simulink model "PID_SMC_for_Hexa_rotor"  (R2021a)
settings: Solver=VariableStepAuto  StartTime=0.0  StopTime=T_s+30  RelTol=1e-3
StartFcn:
  | run('Linearized_model.m')
values from neighbouring files (symbols this model uses):
  a_x = x(1,1:(length(x)-1))    [Linearized_model.m]    (also in Linearized_model_motor_dynamics.m)
  a_y = y(1,1:(length(y)-1))    [Linearized_model.m]    (also in Linearized_model_motor_dynamics.m)
  a_z = z(1,1:(length(z)-1))    [Linearized_model.m]    (also in Linearized_model_motor_dynamics.m)
  b_x = x(1,2:length(x))    [Linearized_model.m]    (also in Linearized_model_motor_dynamics.m)
  b_y = y(1,2:length(y))    [Linearized_model.m]    (also in Linearized_model_motor_dynamics.m)
  b_z = z(1,2:length(z))    [Linearized_model.m]    (also in Linearized_model_motor_dynamics.m)
  T_r = zeros(1, length(T))    [Linearized_model.m]    (also in Linearized_model_motor_dynamics.m)
  T_s = sum(T)    [Linearized_model.m]    (also in Linearized_model_motor_dynamics.m)
undefined symbols (not defined in the file or in its folder): a_phi, a_si, a_theta, b_phi, b_si, b_theta
libraries: sharedtransform x1, uavutilslib x1
settings Model: Creator=Traveler  LastModifiedBy=Traveler

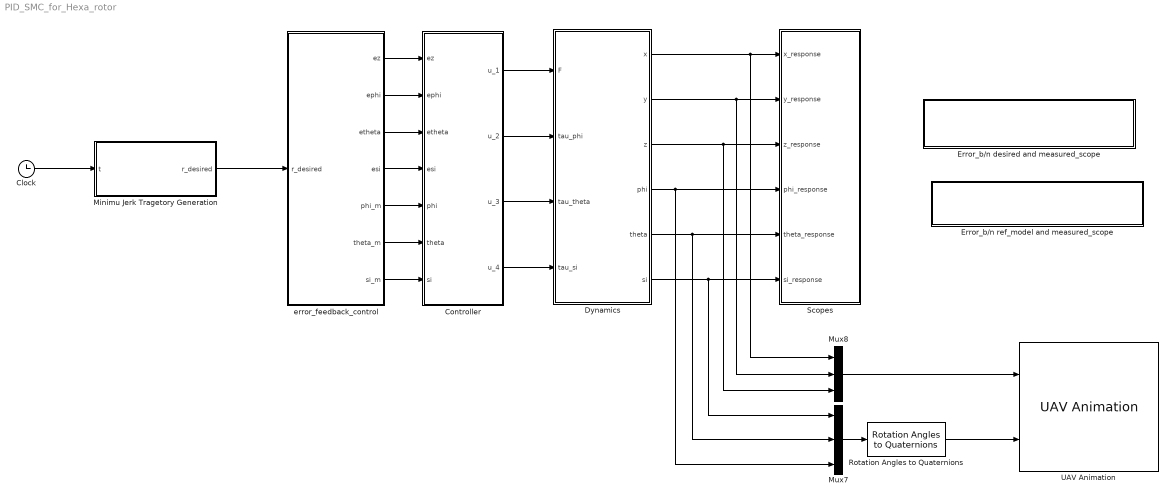
== system PID_SMC_for_Hexa_rotor ==
  Clock : Clock
  Controller : Subsystem
  Dynamics : Subsystem
  Error_b/n desired and measured_scope : Subsystem
  Error_b/n ref_model and measured_scope : Subsystem
  Minimu Jerk Tragetory Generation : Subsystem
  Mux7 : Mux  Inputs=3
  Mux8 : Mux  Inputs=3
  Rotation Angles to Quaternions : sharedtransform/Rotation Angles to Quaternions  rotationOrder=ZYX  aMode=aMode
      settings: SourceProductBaseCode=AE,PW,DR,MT,UV,VE
  Scopes : Subsystem
  UAV Animation : uavutilslib/UAV Animation  UAVType=Multirotor  UAVSize=0.1  InertialZDirection=Up  SampleTime=0.1
      settings: SourceProductBaseCode=UV
  error_feedback_control : Subsystem
  wires:
  error_feedback_control/1(ez) -> Controller/1(ez)
  error_feedback_control/7(si_m) -> Controller/7(si)
  Controller/1(u_1) -> Dynamics/1(F)
  error_feedback_control/2(ephi) -> Controller/2(ephi)
  error_feedback_control/6(theta_m) -> Controller/6(theta)
  error_feedback_control/4(esi) -> Controller/4(esi)
  Clock/1 -> Minimu Jerk Tragetory Generation/1(t)
  error_feedback_control/3(etheta) -> Controller/3(etheta)
  error_feedback_control/5(phi_m) -> Controller/5(phi)
  Controller/2(u_2) -> Dynamics/2(tau_phi)
  Controller/4(u_4) -> Dynamics/4(tau_si)
  Controller/3(u_3) -> Dynamics/3(tau_theta)
  Minimu Jerk Tragetory Generation/1(r_desired) -> error_feedback_control/1(r_desired)
  Rotation Angles to Quaternions/1 -> UAV Animation/2
  Dynamics/2(y) -> Mux8/2, Scopes/2(y_response)
  Mux7/1 -> Rotation Angles to Quaternions/1
  Dynamics/6(si) -> Mux7/1, Scopes/6(si_response)
  Dynamics/1(x) -> Mux8/1, Scopes/1(x_response)
  Dynamics/5(theta) -> Mux7/2, Scopes/5(theta_response)
  Dynamics/3(z) -> Mux8/3, Scopes/3(z_response)
  Dynamics/4(phi) -> Mux7/3, Scopes/4(phi_response)
  Mux8/1 -> UAV Animation/1

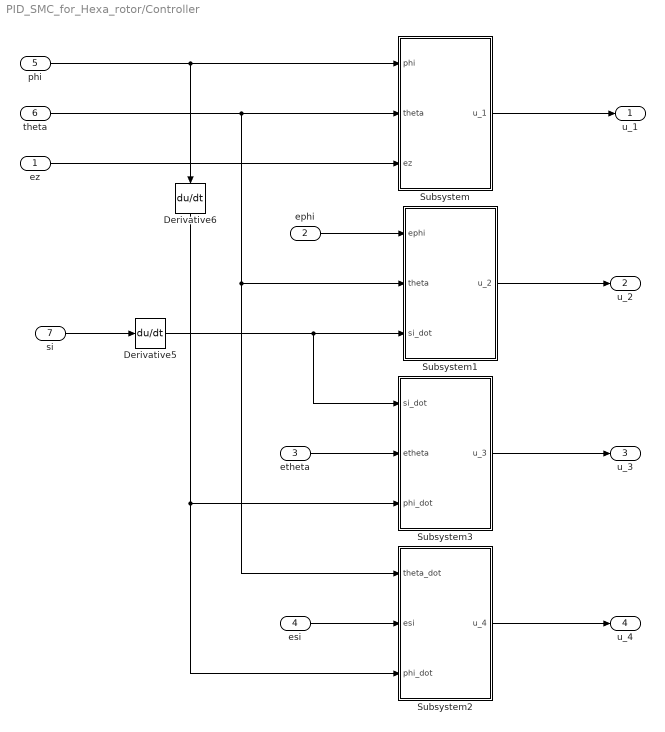
== system PID_SMC_for_Hexa_rotor/Controller ==
  ez : Inport
  ephi : Inport  Port=2
  etheta : Inport  Port=3
  esi : Inport  Port=4
  phi : Inport  Port=5
  theta : Inport  Port=6
  si : Inport  Port=7
  Derivative5 : Derivative
  Derivative6 : Derivative
  Subsystem : Subsystem
  Subsystem1 : Subsystem
  Subsystem2 : Subsystem
  Subsystem3 : Subsystem
  u_1 : Outport
  u_2 : Outport  Port=2
  u_3 : Outport  Port=3
  u_4 : Outport  Port=4
  wires:
  phi/1 -> Derivative6/1, Subsystem/1(phi)
  theta/1 -> Subsystem2/1(theta_dot), Subsystem1/2(theta), Subsystem/2(theta)
  Derivative5/1 -> Subsystem1/3(si_dot), Subsystem3/1(si_dot)
  Derivative6/1 -> Subsystem2/3(phi_dot), Subsystem3/3(phi_dot)
  si/1 -> Derivative5/1
  ez/1 -> Subsystem/3(ez)
  Subsystem/1(u_1) -> u_1/1
  ephi/1 -> Subsystem1/1(ephi)
  Subsystem1/1(u_2) -> u_2/1
  esi/1 -> Subsystem2/2(esi)
  Subsystem2/1(u_4) -> u_4/1
  etheta/1 -> Subsystem3/2(etheta)
  Subsystem3/1(u_3) -> u_3/1

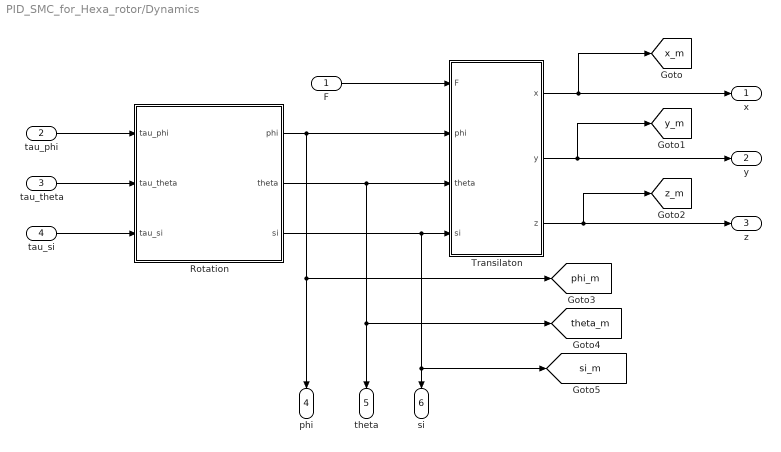
== system PID_SMC_for_Hexa_rotor/Dynamics ==
  F : Inport
  tau_phi : Inport  Port=2
  tau_theta : Inport  Port=3
  tau_si : Inport  Port=4
  Rotation : Subsystem
  Transilaton : Subsystem
  x : Outport
  y : Outport  Port=2
  z : Outport  Port=3
  phi : Outport  Port=4
  theta : Outport  Port=5
  si : Outport  Port=6
  tag scope: phi_m=global, si_m=global, theta_m=global, x_m=global, y_m=global, z_m=global
  wires:
  Transilaton/2(y) -> [y_m], y/1
  Transilaton/1(x) -> [x_m], x/1
  Transilaton/3(z) -> [z_m], z/1
  Rotation/1(phi) -> Transilaton/2(phi), phi/1, [phi_m]
  Rotation/2(theta) -> Transilaton/3(theta), theta/1, [theta_m]
  Rotation/3(si) -> Transilaton/4(si), [si_m], si/1
  tau_phi/1 -> Rotation/1(tau_phi)
  tau_theta/1 -> Rotation/2(tau_theta)
  tau_si/1 -> Rotation/3(tau_si)
  F/1 -> Transilaton/1(F)

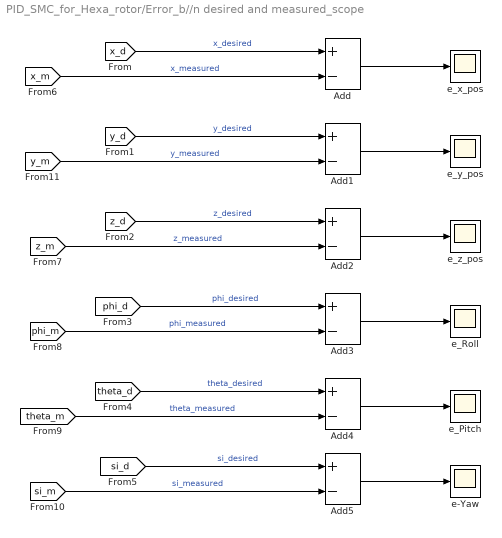
== system PID_SMC_for_Hexa_rotor/Error_b//n desired and measured_scope ==
  Add{,1..5} (6 alike) : Sum  Inputs=+-
  e-Yaw : Scope
  e_Pitch : Scope
  e_Roll : Scope
  e_x_pos : Scope
  e_y_pos : Scope
  e_z_pos : Scope
  wires:
  [x_m] -> Add/2  "x_measured"
  Add/1 -> e_x_pos/1
  [x_d] -> Add/1  "x_desired"
  [y_d] -> Add1/1  "y_desired"
  Add1/1 -> e_y_pos/1
  [z_m] -> Add2/2  "z_measured"
  [z_d] -> Add2/1  "z_desired"
  [phi_d] -> Add3/1  "phi_desired"
  [phi_m] -> Add3/2  "phi_measured"
  [theta_m] -> Add4/2  "theta_measured"
  [theta_d] -> Add4/1  "theta_desired"
  [si_d] -> Add5/1  "si_desired"
  [si_m] -> Add5/2  "si_measured"
  Add2/1 -> e_z_pos/1
  [y_m] -> Add1/2  "y_measured"
  Add5/1 -> e-Yaw/1
  Add3/1 -> e_Roll/1
  Add4/1 -> e_Pitch/1

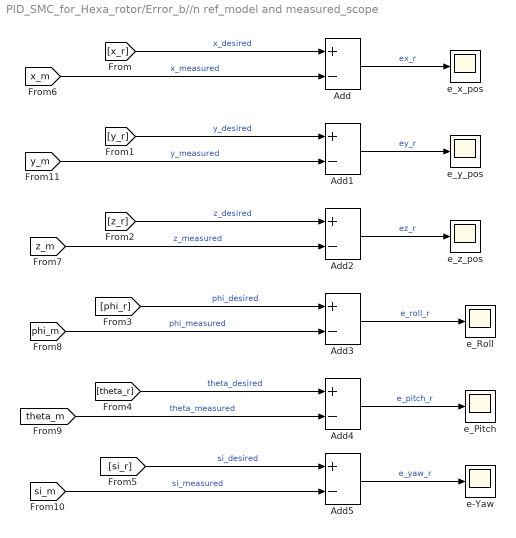
== system PID_SMC_for_Hexa_rotor/Error_b//n ref_model and measured_scope ==
  Add{,1..5} (6 alike) : Sum  Inputs=+-
  e-Yaw : Scope
  e_Pitch : Scope
  e_Roll : Scope
  e_x_pos : Scope
  e_y_pos : Scope
  e_z_pos : Scope
  wires:
  Add4/1 -> e_Pitch/1  "e_pitch_r"
  Add3/1 -> e_Roll/1  "e_roll_r"
  Add5/1 -> e-Yaw/1  "e_yaw_r"
  [y_m] -> Add1/2  "y_measured"
  Add2/1 -> e_z_pos/1  "ez_r"
  [si_m] -> Add5/2  "si_measured"
  [si_r] -> Add5/1  "si_desired"
  [theta_r] -> Add4/1  "theta_desired"
  [theta_m] -> Add4/2  "theta_measured"
  [phi_m] -> Add3/2  "phi_measured"
  [phi_r] -> Add3/1  "phi_desired"
  [z_r] -> Add2/1  "z_desired"
  [z_m] -> Add2/2  "z_measured"
  Add1/1 -> e_y_pos/1  "ey_r"
  [y_r] -> Add1/1  "y_desired"
  [x_r] -> Add/1  "x_desired"
  Add/1 -> e_x_pos/1  "ex_r"
  [x_m] -> Add/2  "x_measured"

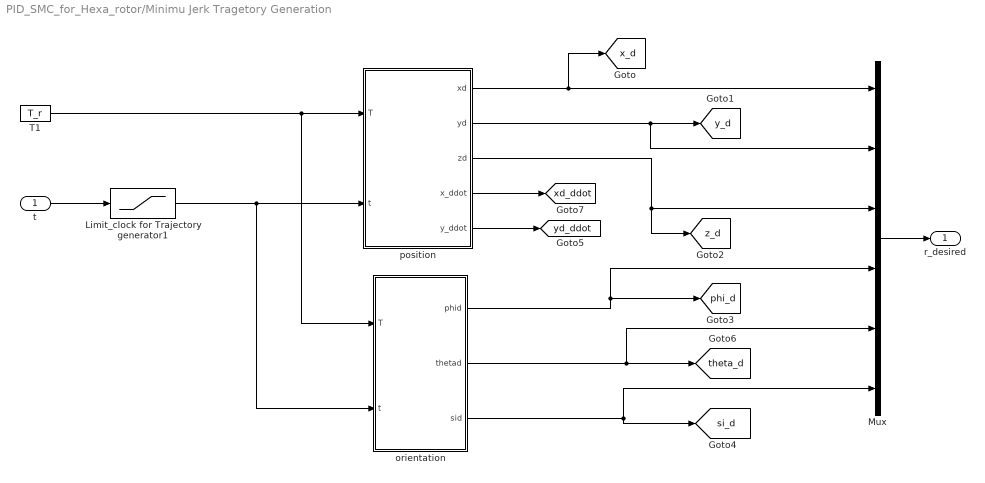
== system PID_SMC_for_Hexa_rotor/Minimu Jerk Tragetory Generation ==
  t : Inport
  Limit_clock for Trajectory generator1 : Saturate  UpperLimit=T_s  LowerLimit=0
  Mux : Mux  Inputs=6
  T1 : Constant  Value=T_r
  orientation : Subsystem
  position : Subsystem
  r_desired : Outport
  tag scope: phi_d=global, si_d=global, theta_d=global, x_d=global, xd_ddot=global, y_d=global, yd_ddot=global, z_d=global
  wires:
  Mux/1 -> r_desired/1
  orientation/1(phid) -> Mux/4, [phi_d]
  orientation/3(sid) -> [si_d], Mux/6
  position/4(x_ddot) -> [xd_ddot]
  position/1(xd) -> Mux/1, [x_d]
  position/3(zd) -> Mux/3, [z_d]
  Limit_clock for Trajectory generator1/1 -> position/2(t), orientation/2(t)
  T1/1 -> position/1(T), orientation/1(T)
  position/5(y_ddot) -> [yd_ddot]
  t/1 -> Limit_clock for Trajectory generator1/1
  orientation/2(thetad) -> Mux/5, [theta_d]
  position/2(yd) -> Mux/2, [y_d]

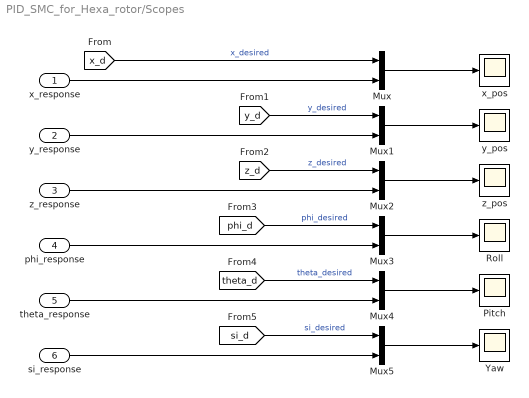
== system PID_SMC_for_Hexa_rotor/Scopes ==
  x_response : Inport
  y_response : Inport  Port=2
  z_response : Inport  Port=3
  phi_response : Inport  Port=4
  theta_response : Inport  Port=5
  si_response : Inport  Port=6
  Mux{,1..5} (6 alike) : Mux  Inputs=2
  Pitch : Scope
  Roll : Scope
  Yaw : Scope
  x_pos : Scope
  y_pos : Scope
  z_pos : Scope
  wires:
  [x_d] -> Mux/1  "x_desired"
  Mux4/1 -> Pitch/1
  [phi_d] -> Mux3/1  "phi_desired"
  Mux2/1 -> z_pos/1
  [si_d] -> Mux5/1  "si_desired"
  [y_d] -> Mux1/1  "y_desired"
  [theta_d] -> Mux4/1  "theta_desired"
  Mux5/1 -> Yaw/1
  Mux/1 -> x_pos/1
  [z_d] -> Mux2/1  "z_desired"
  Mux3/1 -> Roll/1
  y_response/1 -> Mux1/2
  Mux1/1 -> y_pos/1
  theta_response/1 -> Mux4/2
  z_response/1 -> Mux2/2
  phi_response/1 -> Mux3/2
  si_response/1 -> Mux5/2
  x_response/1 -> Mux/2

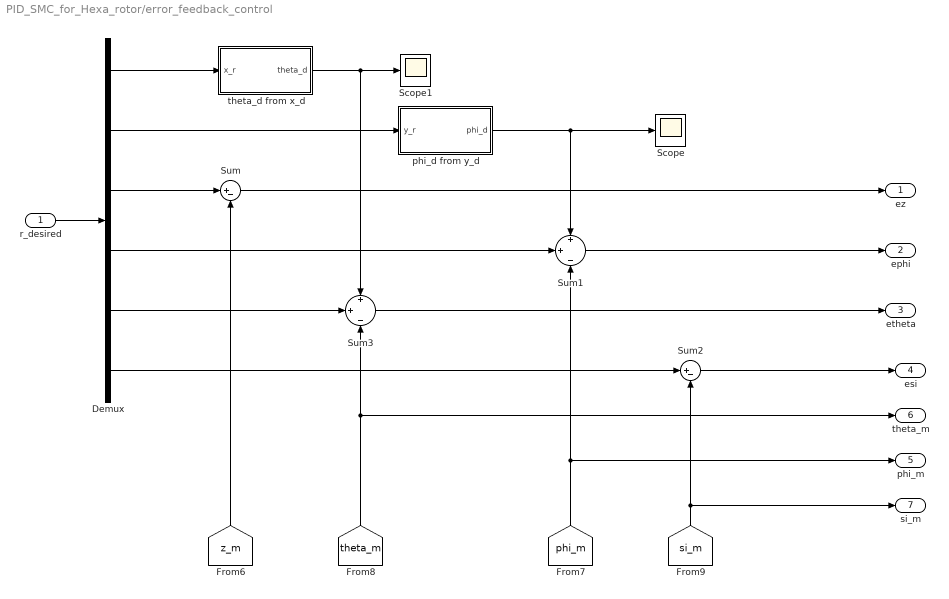
== system PID_SMC_for_Hexa_rotor/error_feedback_control ==
  r_desired : Inport
  Demux : Demux  Outputs=6
  Scope : Scope
  Scope1 : Scope
  Sum : Sum  Inputs=|+-
  Sum1 : Sum  Inputs=+|+|-
  Sum2 : Sum  Inputs=|+-
  Sum3 : Sum  Inputs=+|+|-
  phi_d from y_d : Subsystem
  theta_d from x_d : Subsystem
  ez : Outport
  ephi : Outport  Port=2
  etheta : Outport  Port=3
  esi : Outport  Port=4
  phi_m : Outport  Port=5
  theta_m : Outport  Port=6
  si_m : Outport  Port=7
  wires:
  [theta_m] -> Sum3/3, theta_m/1
  Demux/5 -> Sum3/2
  [phi_m] -> Sum1/3, phi_m/1
  [si_m] -> si_m/1, Sum2/2
  Demux/6 -> Sum2/1
  [z_m] -> Sum/2
  Demux/3 -> Sum/1
  Sum1/1 -> ephi/1
  Sum3/1 -> etheta/1
  Sum/1 -> ez/1
  Sum2/1 -> esi/1
  r_desired/1 -> Demux/1
  Demux/1 -> theta_d from x_d/1(x_r)
  Demux/2 -> phi_d from y_d/1(y_r)
  Demux/4 -> Sum1/2
  phi_d from y_d/1(phi_d) -> Scope/1, Sum1/1
  theta_d from x_d/1(theta_d) -> Sum3/1, Scope1/1

== system PID_SMC_for_Hexa_rotor/Controller/Subsystem ==
  phi : Inport
  theta : Inport  Port=2
  ez : Inport  Port=3
  Derivative : Derivative
  Integrator : Integrator
  Integrator4 : Integrator
  Sliding Mode controller : MATLAB Function  TreatAsAtomicUnit=on
  u_1 : Outport
  wires:
  ez/1 -> Integrator4/1, Derivative/1, Sliding Mode controller/3(ez)
  Integrator4/1 -> Sliding Mode controller/5(ez_int)
  Sliding Mode controller/2(del_hat_dot) -> Integrator/1
  Derivative/1 -> Sliding Mode controller/4(ez_dot)
  Integrator/1 -> Sliding Mode controller/6(del_hat)
  Sliding Mode controller/1(u_1) -> u_1/1
  phi/1 -> Sliding Mode controller/1(phi)
  theta/1 -> Sliding Mode controller/2(theta)

== system PID_SMC_for_Hexa_rotor/Controller/Subsystem1 ==
  ephi : Inport
  theta : Inport  Port=2
  si_dot : Inport  Port=3
  Derivative1 : Derivative
  Derivative4 : Derivative
  Integrator3 : Integrator
  Integrator5 : Integrator
  Sliding Mode controller1 : MATLAB Function  TreatAsAtomicUnit=on
  u_2 : Outport
  wires:
  Sliding Mode controller1/2(del_hat_dot) -> Integrator3/1
  ephi/1 -> Integrator5/1, Derivative1/1, Sliding Mode controller1/1(ephi)
  theta/1 -> Derivative4/1
  Derivative1/1 -> Sliding Mode controller1/2(ephi_dot)
  Sliding Mode controller1/1(u_2) -> u_2/1
  Derivative4/1 -> Sliding Mode controller1/4(theta_dot)
  Integrator3/1 -> Sliding Mode controller1/6(del_hat)
  Integrator5/1 -> Sliding Mode controller1/3(ephi_int)
  si_dot/1 -> Sliding Mode controller1/5(si_dot)

== system PID_SMC_for_Hexa_rotor/Controller/Subsystem2 ==
  theta_dot : Inport
  esi : Inport  Port=2
  phi_dot : Inport  Port=3
  Derivative3 : Derivative
  Integrator2 : Integrator
  Integrator7 : Integrator
  Sliding Mode controller3 : MATLAB Function  TreatAsAtomicUnit=on
  u_4 : Outport
  wires:
  theta_dot/1 -> Sliding Mode controller3/4(theta_dot)
  esi/1 -> Sliding Mode controller3/1(esi), Integrator7/1, Derivative3/1
  Derivative3/1 -> Sliding Mode controller3/2(esi_dot)
  Integrator2/1 -> Sliding Mode controller3/6(del_hat)
  Integrator7/1 -> Sliding Mode controller3/3(esi_int)
  Sliding Mode controller3/2(del_hat_dot) -> Integrator2/1
  Sliding Mode controller3/1(u_4) -> u_4/1
  phi_dot/1 -> Sliding Mode controller3/5(phi_dot)

== system PID_SMC_for_Hexa_rotor/Controller/Subsystem3 ==
  si_dot : Inport
  etheta : Inport  Port=2
  phi_dot : Inport  Port=3
  Derivative2 : Derivative
  Integrator1 : Integrator
  Integrator6 : Integrator
  Sliding Mode controller2 : MATLAB Function  TreatAsAtomicUnit=on
  u_3 : Outport
  wires:
  Sliding Mode controller2/2(del_hat_dot) -> Integrator1/1
  Integrator1/1 -> Sliding Mode controller2/6(del_hat)
  Sliding Mode controller2/1(u_3) -> u_3/1
  Integrator6/1 -> Sliding Mode controller2/3(etheta_int)
  etheta/1 -> Sliding Mode controller2/1(etheta), Integrator6/1, Derivative2/1
  Derivative2/1 -> Sliding Mode controller2/2(etheta_dot)
  phi_dot/1 -> Sliding Mode controller2/4(phi_dot)
  si_dot/1 -> Sliding Mode controller2/5(si_dot)

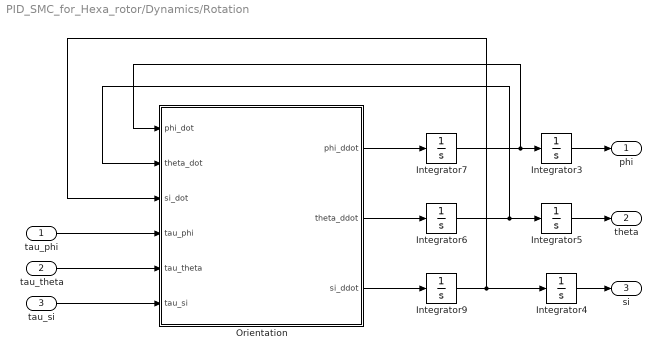
== system PID_SMC_for_Hexa_rotor/Dynamics/Rotation ==
  tau_phi : Inport
  tau_theta : Inport  Port=2
  tau_si : Inport  Port=3
  Integrator{3..7,9} (6 alike) : Integrator
  Orientation : MATLAB Function  TreatAsAtomicUnit=on
  phi : Outport
  theta : Outport  Port=2
  si : Outport  Port=3
  wires:
  Orientation/2(theta_ddot) -> Integrator6/1
  Integrator9/1 -> Orientation/3(si_dot), Integrator4/1
  Orientation/3(si_ddot) -> Integrator9/1
  Orientation/1(phi_ddot) -> Integrator7/1
  Integrator7/1 -> Orientation/1(phi_dot), Integrator3/1
  Integrator6/1 -> Integrator5/1, Orientation/2(theta_dot)
  tau_theta/1 -> Orientation/5(tau_theta)
  tau_phi/1 -> Orientation/4(tau_phi)
  tau_si/1 -> Orientation/6(tau_si)
  Integrator3/1 -> phi/1
  Integrator4/1 -> si/1
  Integrator5/1 -> theta/1

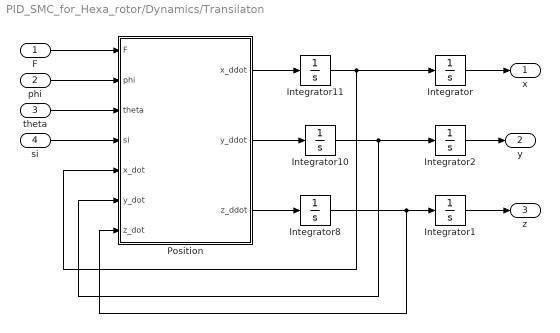
== system PID_SMC_for_Hexa_rotor/Dynamics/Transilaton ==
  F : Inport
  phi : Inport  Port=2
  theta : Inport  Port=3
  si : Inport  Port=4
  Integrator{,1..2,8,10..11} (6 alike) : Integrator
  Position : MATLAB Function  TreatAsAtomicUnit=on
  x : Outport
  y : Outport  Port=2
  z : Outport  Port=3
  wires:
  Integrator8/1 -> Integrator1/1, Position/7(z_dot)
  Position/3(z_ddot) -> Integrator8/1
  phi/1 -> Position/2(phi)
  Integrator10/1 -> Position/6(y_dot), Integrator2/1
  Integrator1/1 -> z/1
  Position/2(y_ddot) -> Integrator10/1
  Position/1(x_ddot) -> Integrator11/1
  Integrator11/1 -> Position/5(x_dot), Integrator/1
  Integrator/1 -> x/1
  Integrator2/1 -> y/1
  si/1 -> Position/4(si)
  theta/1 -> Position/3(theta)
  F/1 -> Position/1(F)

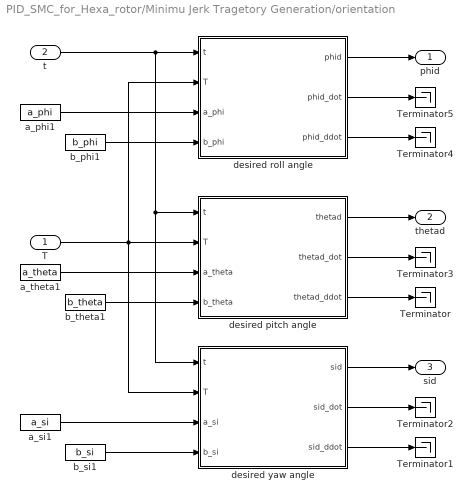
== system PID_SMC_for_Hexa_rotor/Minimu Jerk Tragetory Generation/orientation ==
  T : Inport
  t : Inport  Port=2
  " desired pitch angle" : MATLAB Function  TreatAsAtomicUnit=on
  Terminator{,1..5} (6 alike) : Terminator
  a_phi1 : Constant  Value=a_phi
  a_si1 : Constant  Value=a_si
  a_theta1 : Constant  Value=a_theta
  b_phi1 : Constant  Value=b_phi
  b_si1 : Constant  Value=b_si
  b_theta1 : Constant  Value=b_theta
  desired roll angle : MATLAB Function  TreatAsAtomicUnit=on
  desired yaw angle : MATLAB Function  TreatAsAtomicUnit=on
  phid : Outport
  thetad : Outport  Port=2
  sid : Outport  Port=3
  wires:
  desired roll angle/1(phid) -> phid/1
  desired roll angle/2(phid_dot) -> Terminator5/1
  desired roll angle/3(phid_ddot) -> Terminator4/1
  " desired pitch angle"/3(thetad_ddot) -> Terminator/1
  " desired pitch angle"/2(thetad_dot) -> Terminator3/1
  " desired pitch angle"/1(thetad) -> thetad/1
  desired yaw angle/1(sid) -> sid/1
  desired yaw angle/2(sid_dot) -> Terminator2/1
  desired yaw angle/3(sid_ddot) -> Terminator1/1
  a_phi1/1 -> desired roll angle/3(a_phi)
  b_phi1/1 -> desired roll angle/4(b_phi)
  a_theta1/1 -> " desired pitch angle"/3(a_theta)
  b_theta1/1 -> " desired pitch angle"/4(b_theta)
  a_si1/1 -> desired yaw angle/3(a_si)
  b_si1/1 -> desired yaw angle/4(b_si)
  T/1 -> desired roll angle/2(T), " desired pitch angle"/2(T), desired yaw angle/2(T)
  t/1 -> desired yaw angle/1(t), " desired pitch angle"/1(t), desired roll angle/1(t)

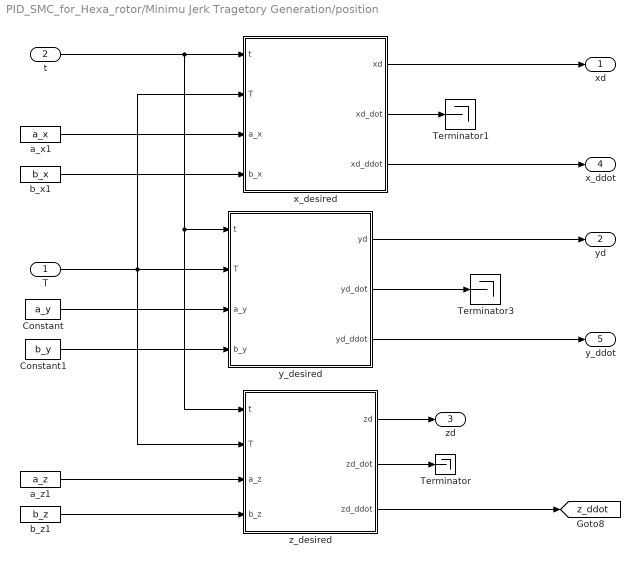
== system PID_SMC_for_Hexa_rotor/Minimu Jerk Tragetory Generation/position ==
  T : Inport
  t : Inport  Port=2
  " z_desired" : MATLAB Function  TreatAsAtomicUnit=on
  Constant : Constant  Value=a_y
  Constant1 : Constant  Value=b_y
  Terminator : Terminator
  Terminator1 : Terminator
  Terminator3 : Terminator
  a_x1 : Constant  Value=a_x
  a_z1 : Constant  Value=a_z
  b_x1 : Constant  Value=b_x
  b_z1 : Constant  Value=b_z
  x_desired : MATLAB Function  TreatAsAtomicUnit=on
  y_desired : MATLAB Function  TreatAsAtomicUnit=on
  xd : Outport
  yd : Outport  Port=2
  zd : Outport  Port=3
  x_ddot : Outport  Port=4
  y_ddot : Outport  Port=5
  tag scope: z_ddot=global
  wires:
  y_desired/1(yd) -> yd/1
  T/1 -> x_desired/2(T), y_desired/2(T), " z_desired"/2(T)
  a_x1/1 -> x_desired/3(a_x)
  b_x1/1 -> x_desired/4(b_x)
  Constant/1 -> y_desired/3(a_y)
  Constant1/1 -> y_desired/4(b_y)
  a_z1/1 -> " z_desired"/3(a_z)
  b_z1/1 -> " z_desired"/4(b_z)
  " z_desired"/2(zd_dot) -> Terminator/1
  x_desired/2(xd_dot) -> Terminator1/1
  y_desired/2(yd_dot) -> Terminator3/1
  t/1 -> x_desired/1(t), y_desired/1(t), " z_desired"/1(t)
  " z_desired"/3(zd_ddot) -> [z_ddot]
  " z_desired"/1(zd) -> zd/1
  y_desired/3(yd_ddot) -> y_ddot/1
  x_desired/3(xd_ddot) -> x_ddot/1
  x_desired/1(xd) -> xd/1

== system PID_SMC_for_Hexa_rotor/error_feedback_control/phi_d from y_d ==
  y_r : Inport
  Derivative1 : Derivative
  Integrator1 : Integrator
  Integrator2 : Integrator  InitialCondition=0.1
  MATLAB Function : MATLAB Function  TreatAsAtomicUnit=on
  Sum : Sum  Inputs=|+-
  phi_d : Outport
  wires:
  MATLAB Function/1(phi_d) -> phi_d/1
  [y_m] -> Sum/2
  y_r/1 -> Sum/1
  Integrator2/1 -> MATLAB Function/5(gm)
  [yd_ddot] -> MATLAB Function/1(yd_ddot)
  MATLAB Function/2(gm_dot) -> Integrator2/1
  Integrator1/1 -> MATLAB Function/3(ey_int)
  Derivative1/1 -> MATLAB Function/4(ey_dot)
  Sum/1 -> Derivative1/1, Integrator1/1, MATLAB Function/2(ey)

== system PID_SMC_for_Hexa_rotor/error_feedback_control/theta_d from x_d ==
  x_r : Inport
  Derivative : Derivative
  Integrator : Integrator
  Integrator1 : Integrator  InitialCondition=0.1
  MATLAB Function1 : MATLAB Function  TreatAsAtomicUnit=on
  Sum : Sum  Inputs=|+-
  theta_d : Outport
  wires:
  x_r/1 -> Sum/1
  [x_m] -> Sum/2
  Integrator1/1 -> MATLAB Function1/5(gm)
  MATLAB Function1/2(gm_dot) -> Integrator1/1
  [xd_ddot] -> MATLAB Function1/1(xd_ddot)
  Sum/1 -> Derivative/1, Integrator/1, MATLAB Function1/2(ex)
  Integrator/1 -> MATLAB Function1/3(ex_int)
  Derivative/1 -> MATLAB Function1/4(ex_dot)
  MATLAB Function1/1(theta_d) -> theta_d/1

== matlab function PID_SMC_for_Hexa_rotor/Dynamics/Rotation/Orientation ==
  data: phi_dot input; theta_dot input; si_dot input; tau_phi input; tau_theta input; tau_si input; phi_ddot output; theta_ddot output; si_ddot output
function [phi_ddot,theta_ddot,si_ddot] = fcn(phi_dot,theta_dot,si_dot,tau_phi, tau_theta, tau_si)
[Jx,Jy,Jz]=deal(0.01);
k_phi=0.1;
k_theta=0.1;
k_si=0.1;
Jr=0.025;
omega_r=0.025;
phi_ddot= (theta_dot* si_dot*(Jy - Jz) - k_phi*phi_dot^2 - Jr*omega_r*theta_dot + tau_phi)/Jx;
theta_ddot=(phi_dot* si_dot*(Jz - Jx)  - k_theta*theta_dot^2 + Jr*omega_r*phi_dot + tau_theta)/Jy;
si_ddot=(phi_dot* theta_dot*(Jy - Jz) - k_si*si_dot^2 + tau_si)/Jz;
end

== matlab function PID_SMC_for_Hexa_rotor/Minimu Jerk Tragetory Generation/orientation/desired yaw angle ==
  data: t input; T input; sid output; sid_dot output; sid_ddot output; a_si input; b_si input
function [sid,sid_dot,sid_ddot] = fcn(t,T,a_si,b_si)
T0 = 0; % Initialize T0
Tf = 0; % Initialize Tf
a = 0;  % Initialize a
b = 0;  % Initialize b

for i = 1:length(T)
    if (i == 1 && t <= T(i))
        Tf = T(i);
        a = a_si(i);
        b = b_si(i);
        break;
    elseif (i > 1 && t > T(i-1) && t <= T(i))
        T0 = T(i-1);
        Tf = T(i);
        a = a_si(i);
        b = b_si(i);
        break;
    end
end
if (t > T(end-1)) % Handle the case where t is greater than the last interval
    T0 = T(end-1);
    Tf = T(end);
    a = a_si(end);
    b = b_si(end);
end
B=[a;b;0;0;0;0];
A=[T0^5     T0^4     T0^3    T0^2  T0^1  1;
   Tf^5     Tf^4     Tf^3    Tf^2  Tf^1  1;
   5*T0^4   4*T0^3   3*T0^2  2*T0  1     0;
   5*Tf^4   4*Tf^3   3*Tf^2  2*Tf  1     0;
   20*T0^3  12*T0^2  6*T0    2     0     0;
   20*Tf^3  12*Tf^2  6*Tf    2     0     0];
C=A\B;
sid=C(1,1)*t^5 + C(2,1)*t^4 + C(3,1)*t^3 + C(4,1)*t^2 + C(5,1)*t + C(6,1);
sid_dot=5*C(1,1)*t^4  + 4*C(2,1)*t^3 + 3*C(3,1)*t^2 + 2*C(4,1)*t + C(5,1);
sid_ddot=20*C(1,1)*t^3  + 12*C(2,1)*t^2 + 6*C(3,1)*t + 2*C(4,1);
end

== matlab function PID_SMC_for_Hexa_rotor/Minimu Jerk Tragetory Generation/position/ z_desired ==
  data: t input; T input; zd output; zd_dot output; zd_ddot output; a_z input; b_z input
function [zd,zd_dot,zd_ddot] = fcn(t,T,a_z,b_z)
T0 = 0; % Initialize T0
Tf = 0; % Initialize Tf
a = 0;  % Initialize a
b = 0;  % Initialize b

for i = 1:length(T)
    if (i == 1 && t <= T(i))
        Tf = T(i);
        a = a_z(i);
        b = b_z(i);
        break;
    elseif (i > 1 && t > T(i-1) && t <= T(i))
        T0 = T(i-1);
        Tf = T(i);
        a = a_z(i);
        b = b_z(i);
        break;
    end
end
if (t > T(end-1)) % Handle the case where t is greater than the last interval
    T0 = T(end-1);
    Tf = T(end);
    a = a_z(end);
    b = b_z(end);
end
B=[a;b;0;0;0;0];
A=[T0^5     T0^4     T0^3    T0^2  T0^1  1;
   Tf^5     Tf^4     Tf^3    Tf^2  Tf^1  1;
   5*T0^4   4*T0^3   3*T0^2  2*T0  1     0;
   5*Tf^4   4*Tf^3   3*Tf^2  2*Tf  1     0;
   20*T0^3  12*T0^2  6*T0    2     0     0;
   20*Tf^3  12*Tf^2  6*Tf    2     0     0];
C=A\B;
zd=C(1,1)*t^5 + C(2,1)*t^4 + C(3,1)*t^3 + C(4,1)*t^2 + C(5,1)*t + C(6,1);
zd_dot=5*C(1,1)*t^4  + 4*C(2,1)*t^3 + 3*C(3,1)*t^2 + 2*C(4,1)*t + C(5,1);
zd_ddot=20*C(1,1)*t^3  + 12*C(2,1)*t^2 + 6*C(3,1)*t + 2*C(4,1);
end

== matlab function PID_SMC_for_Hexa_rotor/Minimu Jerk Tragetory Generation/position/x_desired ==
  data: t input; T input; xd output; xd_dot output; xd_ddot output; a_x input; b_x input
function [xd,xd_dot,xd_ddot] = fcn(t,T,a_x,b_x)
T0 = 0; % Initialize T0
Tf = 0; % Initialize Tf
a = 0;  % Initialize a
b = 0;  % Initialize b

for i = 1:length(T)
    if (i == 1 && t <= T(i))
        Tf = T(i);
        a = a_x(i);
        b = b_x(i);
        break;
    elseif (i > 1 && t > T(i-1) && t <= T(i))
        T0 = T(i-1);
        Tf = T(i);
        a = a_x(i);
        b = b_x(i);
        break;
    end
end
if (t > T(end-1)) % Handle the case where t is greater than the last interval
    T0 = T(end-1);
    Tf = T(end);
    a = a_x(end);
    b = b_x(end);
end
B=[a;b;0;0;0;0];
A=[T0^5     T0^4     T0^3    T0^2  T0^1  1;
   Tf^5     Tf^4     Tf^3    Tf^2  Tf^1  1;
   5*T0^4   4*T0^3   3*T0^2  2*T0  1     0;
   5*Tf^4   4*Tf^3   3*Tf^2  2*Tf  1     0;
   20*T0^3  12*T0^2  6*T0    2     0     0;
   20*Tf^3  12*Tf^2  6*Tf    2     0     0];
C=A\B;
xd=C(1,1)*t^5 + C(2,1)*t^4 + C(3,1)*t^3 + C(4,1)*t^2 + C(5,1)*t + C(6,1);
xd_dot=5*C(1,1)*t^4  + 4*C(2,1)*t^3 + 3*C(3,1)*t^2 + 2*C(4,1)*t + C(5,1);
xd_ddot=20*C(1,1)*t^3  + 12*C(2,1)*t^2 + 6*C(3,1)*t + 2*C(4,1);
end

== matlab function PID_SMC_for_Hexa_rotor/Minimu Jerk Tragetory Generation/position/y_desired ==
  data: t input; T input; yd output; yd_dot output; yd_ddot output; a_y input; b_y input
function [yd,yd_dot,yd_ddot] = fcn(t,T,a_y,b_y)
T0 = 0; % Initialize T0
Tf = 0; % Initialize Tf
a = 0;  % Initialize a
b = 0;  % Initialize b

for i = 1:length(T)
    if (i == 1 && t <= T(i))
        Tf = T(i);
        a = a_y(i);
        b = b_y(i);
        break;
    elseif (i > 1 && t > T(i-1) && t <= T(i))
        T0 = T(i-1);
        Tf = T(i);
        a = a_y(i);
        b = b_y(i);
        break;
    end
end
if (t > T(end-1)) % Handle the case where t is greater than the last interval
    T0 = T(end-1);
    Tf = T(end);
    a = a_y(end);
    b = b_y(end);
end
B=[a;b;0;0;0;0];
A=[T0^5     T0^4     T0^3    T0^2  T0^1  1;
   Tf^5     Tf^4     Tf^3    Tf^2  Tf^1  1;
   5*T0^4   4*T0^3   3*T0^2  2*T0  1     0;
   5*Tf^4   4*Tf^3   3*Tf^2  2*Tf  1     0;
   20*T0^3  12*T0^2  6*T0    2     0     0;
   20*Tf^3  12*Tf^2  6*Tf    2     0     0];
C=A\B;
yd=C(1,1)*t^5 + C(2,1)*t^4 + C(3,1)*t^3 + C(4,1)*t^2 + C(5,1)*t + C(6,1);
yd_dot=5*C(1,1)*t^4  + 4*C(2,1)*t^3 + 3*C(3,1)*t^2 + 2*C(4,1)*t + C(5,1);
yd_ddot=20*C(1,1)*t^3  + 12*C(2,1)*t^2 + 6*C(3,1)*t + 2*C(4,1);
end

== matlab function PID_SMC_for_Hexa_rotor/Controller/Subsystem3/Sliding Mode controller2 ==
  data: etheta input; etheta_dot input; etheta_int input; phi_dot input; si_dot input; del_hat input; u_3 output; del_hat_dot output
function [u_3,del_hat_dot] = fcn(etheta,etheta_dot,etheta_int,phi_dot,si_dot,del_hat)
kp=80; ki=100; kd=2; lamda=0.0001;k=2.5;
% kp=350; ki=4; kd=2; lamda=0.001;k=4.75;
I_xx=0.01;I_yy=0.01;I_zz=0.01;J=0.25;omega=0.025;
s_theta=kp*etheta + ki*etheta_int + kd*etheta_dot;
del_hat_dot=lamda*s_theta;
u_3=I_yy*(k*s_theta - phi_dot*si_dot*(I_zz-I_xx) - J*omega*phi_dot - del_hat);

== matlab function PID_SMC_for_Hexa_rotor/Controller/Subsystem2/Sliding Mode controller3 ==
  data: esi input; esi_dot input; esi_int input; theta_dot input; phi_dot input; del_hat input; u_4 output; del_hat_dot output
function [u_4,del_hat_dot] = fcn(esi, esi_dot,esi_int,theta_dot,phi_dot,del_hat)
% kp=8; ki=10; kd=1; lamda=0.0001;k=2.5;
kp=3.5; ki=4; kd=2; lamda=0.001;k=4.75;
I_xx=0.1;I_yy=0.1;I_zz=0.1;
s_theta=kp*esi + ki*esi_int + kd*esi_dot;
del_hat_dot=lamda*s_theta;
u_4=I_zz*(k*s_theta - phi_dot*theta_dot*(I_xx -I_yy) - del_hat);

== matlab function PID_SMC_for_Hexa_rotor/error_feedback_control/phi_d from y_d/MATLAB Function ==
  data: phi_d output; yd_ddot input; ey input; ey_int input; ey_dot input; gm_dot output; gm input
function [phi_d,gm_dot]= fcn(yd_ddot,ey,ey_int,ey_dot,gm)
m=2.5;g=9.81;
kp=100; ki=0.5; kd =0.01;lamda=0.0001; k=0.00001;
s_y=kp*ey + ki*ey_int + kd*ey_dot;
gm_dot=lamda*s_y;
u_y=m*(yd_ddot + gm*s_y - k*sign(s_y));
phi_d=-asin(u_y/g);

== matlab function PID_SMC_for_Hexa_rotor/error_feedback_control/theta_d from x_d/MATLAB Function1 ==
  data: theta_d output; xd_ddot input; ex input; ex_int input; ex_dot input; gm_dot output; gm input
function [theta_d,gm_dot]= fcn(xd_ddot,ex,ex_int,ex_dot,gm)
m=2.5;g=9.81;
kp=100; ki=0.5; kd=0.01; lamda=0.001; k=0.00001;
s_x=kp*ex + ki*ex_int + kd*ex_dot;
gm_dot=lamda*s_x;
u_x=m*(xd_ddot + gm*s_x - k*sign(s_x));
theta_d=asin(u_x/g);

== matlab function PID_SMC_for_Hexa_rotor/Controller/Subsystem/Sliding Mode controller ==
  data: phi input; u_1 output; theta input; ez input; ez_dot input; ez_int input; del_hat_dot output; del_hat input
function [u_1,del_hat_dot]= fcn(phi,theta,ez,ez_dot,ez_int,del_hat)
kp=350; ki=400; kd=200; lamda=0.001;k=4.75;
g=9.81;
m=6;
s_z=kp*ez + ki*ez_int + kd*ez_dot;
del_hat_dot=lamda*s_z;
u_1=m*(g + k*s_z - del_hat)/(cos(theta)*cos(phi));

== matlab function PID_SMC_for_Hexa_rotor/Controller/Subsystem1/Sliding Mode controller1 ==
  data: ephi input; ephi_dot input; ephi_int input; theta_dot input; si_dot input; del_hat input; u_2 output; del_hat_dot output
function [u_2,del_hat_dot] = fcn(ephi,ephi_dot,ephi_int,theta_dot,si_dot,del_hat)
kp=3500; ki=100; kd=0.2; lamda=0.001;k=0.05;
% kp=3.5; ki=4; kd=2; lamda=0.001;k=4.75;
I_xx=0.1;I_yy=0.1;I_zz=0.1;J=0.0025;omega=0.0025;
s_phi=kp*ephi+ ki*ephi_int + kd*ephi_dot;
del_hat_dot=lamda*s_phi;
u_2=I_xx*(k*s_phi - theta_dot*si_dot*(I_yy-I_zz) + J*omega*theta_dot - del_hat);

== matlab function PID_SMC_for_Hexa_rotor/Minimu Jerk Tragetory Generation/orientation/ desired pitch angle ==
  data: t input; T input; thetad output; thetad_dot output; thetad_ddot output; a_theta input; b_theta input
function [thetad,thetad_dot,thetad_ddot] = fcn(t,T,a_theta,b_theta)
T0 = 0; % Initialize T0
Tf = 0; % Initialize Tf
a = 0;  % Initialize a
b = 0;  % Initialize b

for i = 1:length(T)
    if (i == 1 && t <= T(i))
        Tf = T(i);
        a = a_theta(i);
        b = b_theta(i);
        break;
    elseif (i > 1 && t > T(i-1) && t <= T(i))
        T0 = T(i-1);
        Tf = T(i);
        a = a_theta(i);
        b = b_theta(i);
        break;
    end
end
if (t > T(end-1)) % Handle the case where t is greater than the last interval
    T0 = T(end-1);
    Tf = T(end);
    a = a_theta(end);
    b = b_theta(end);
end
B=[a;b;0;0;0;0];
A=[T0^5     T0^4     T0^3    T0^2  T0^1  1;
   Tf^5     Tf^4     Tf^3    Tf^2  Tf^1  1;
   5*T0^4   4*T0^3   3*T0^2  2*T0  1     0;
   5*Tf^4   4*Tf^3   3*Tf^2  2*Tf  1     0;
   20*T0^3  12*T0^2  6*T0    2     0     0;
   20*Tf^3  12*Tf^2  6*Tf    2     0     0];
C=A\B;
thetad=C(1,1)*t^5 + C(2,1)*t^4 + C(3,1)*t^3 + C(4,1)*t^2 + C(5,1)*t + C(6,1);
thetad_dot=5*C(1,1)*t^4  + 4*C(2,1)*t^3 + 3*C(3,1)*t^2 + 2*C(4,1)*t + C(5,1);
thetad_ddot=20*C(1,1)*t^3  + 12*C(2,1)*t^2 + 6*C(3,1)*t + 2*C(4,1);
end

== matlab function PID_SMC_for_Hexa_rotor/Minimu Jerk Tragetory Generation/orientation/desired roll angle ==
  data: t input; T input; phid output; phid_dot output; phid_ddot output; a_phi input; b_phi input
function [phid,phid_dot,phid_ddot] = fcn(t,T,a_phi,b_phi)
T0 = 0; % Initialize T0
Tf = 0; % Initialize Tf
a = 0;  % Initialize a
b = 0;  % Initialize b

for i = 1:length(T)
    if (i == 1 && t <= T(i))
        Tf = T(i);
        a = a_phi(i);
        b = b_phi(i);
        break;
    elseif (i > 1 && t > T(i-1) && t <= T(i))
        T0 = T(i-1);
        Tf = T(i);
        a = a_phi(i);
        b = b_phi(i);
        break;
    end
end
if (t > T(end-1)) % Handle the case where t is greater than the last interval
    T0 = T(end-1);
    Tf = T(end);
    a = a_phi(end);
    b = b_phi(end);
end
B=[a;b;0;0;0;0];
A=[T0^5     T0^4     T0^3    T0^2  T0^1  1;
   Tf^5     Tf^4     Tf^3    Tf^2  Tf^1  1;
   5*T0^4   4*T0^3   3*T0^2  2*T0  1     0;
   5*Tf^4   4*Tf^3   3*Tf^2  2*Tf  1     0;
   20*T0^3  12*T0^2  6*T0    2     0     0;
   20*Tf^3  12*Tf^2  6*Tf    2     0     0];
C=A\B;
phid=C(1,1)*t^5 + C(2,1)*t^4 + C(3,1)*t^3 + C(4,1)*t^2 + C(5,1)*t + C(6,1);
phid_dot=5*C(1,1)*t^4  + 4*C(2,1)*t^3 + 3*C(3,1)*t^2 + 2*C(4,1)*t + C(5,1);
phid_ddot=20*C(1,1)*t^3  + 12*C(2,1)*t^2 + 6*C(3,1)*t + 2*C(4,1);
end

== matlab function PID_SMC_for_Hexa_rotor/Dynamics/Transilaton/Position ==
  data: F input; phi input; theta input; x_ddot output; y_ddot output; z_ddot output; si input; x_dot input; y_dot input; z_dot input
function [x_ddot,y_ddot,z_ddot] = fcn(F,phi,theta,si,x_dot,y_dot,z_dot)
m=6;
g=9.81;
kx=2.5;
ky=2.1;
kz=2.9;
x_ddot=(cos(phi)*sin(theta)*cos(si) + sin(phi)*sin(si))*F/m - kx*x_dot/m;
y_ddot=(cos(phi)*sin(theta)*sin(si) - sin(phi)*cos(si))*F/m - ky*y_dot/m;
z_ddot=-g + cos(phi)*cos(theta)*F/m - kz*z_dot/m;
end
